simulink model "Simulink3"  (R2023b)
settings: Solver=VariableStepAuto  StartTime=0.0  StopTime=10.0  RelTol=1e-3
values from neighbouring files (symbols this model uses):
  x1 = vX1(j)    [call_RTO.m]    (also in modelSolve.m = par(2); modelSolve1.m = par(2))
  x2 = x(2)    [modelSolve.m]    (also in modelSolve1.m)
  x4 = x(4)    [modelSolve.m]    (also in modelSolve1.m)
undefined symbols (not defined in the file or in its folder): x5, x6
settings Model: Creator=bjark  LastModifiedBy=bjark

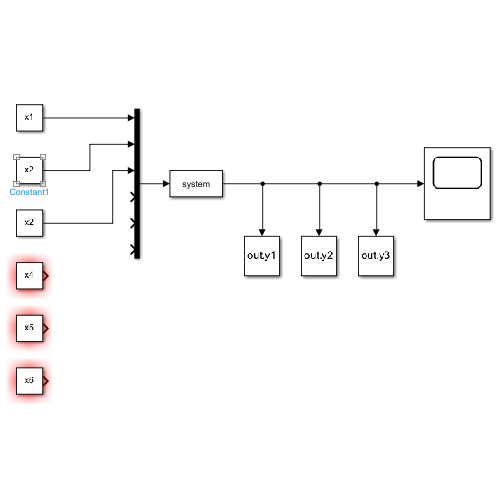
[thumbnail: Simulink's stored preview of the top-level diagram]
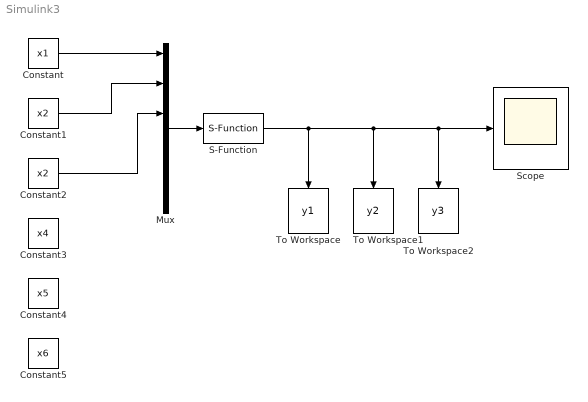
== system Simulink3 ==
  Constant : Constant  Value=x1
  Constant1 : Constant  Value=x2
  Constant2 : Constant  Value=x2
  Constant3 : Constant  Value=x4
  Constant4 : Constant  Value=x5
  Constant5 : Constant  Value=x6
  Mux : Mux  Inputs=6
  S-Function : S-Function  SFunctionDeploymentMode=off  EnableBusSupport=off
  Scope : Scope
  To Workspace : ToWorkspace  VariableName=y1  SampleTime=-1
  To Workspace1 : ToWorkspace  VariableName=y2  SampleTime=-1
  To Workspace2 : ToWorkspace  VariableName=y3  SampleTime=-1
  wires:
  Constant/1 -> Mux/1
  Constant1/1 -> Mux/2
  Constant2/1 -> Mux/3
  Mux/1 -> S-Function/1
  S-Function/1 -> To Workspace/1, Scope/1, To Workspace2/1, To Workspace1/1
